simulink model "Sim48"  (R2019a)
settings: Solver=FixedStepAuto  StartTime=0.0  StopTime=10.0  FixedStep=0.0001  RelTol=1e-3
settings Model: Creator=fbleo  LastModifiedBy=fbleo

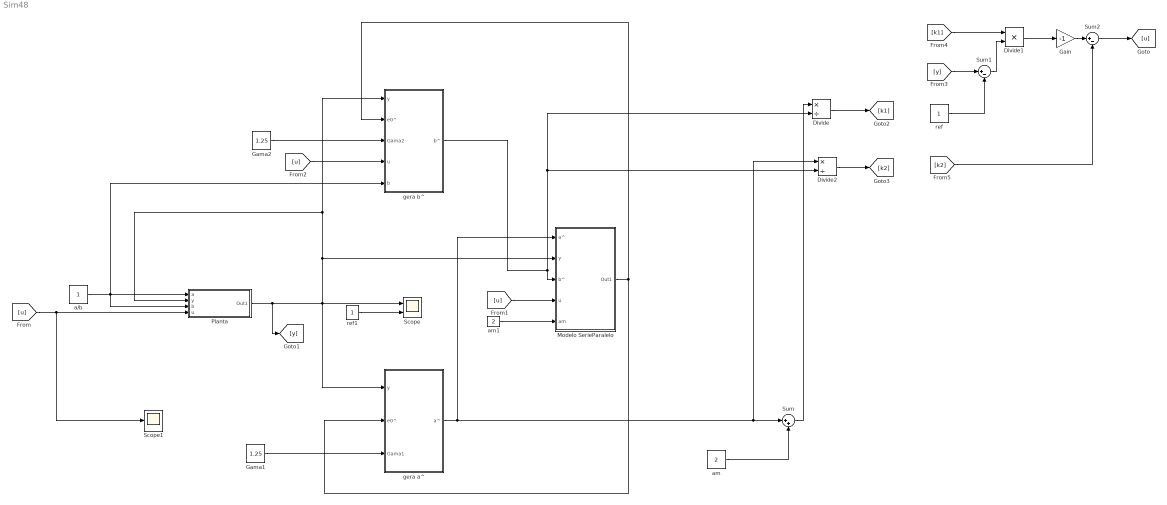
== system Sim48 ==
  Divide : Product  Inputs=*/
  Divide1 : Product  Inputs=**
  Divide2 : Product  Inputs=*/
  Gain : Gain  Gain=-1
  Gama1 : Constant  Value=1.25
  Gama2 : Constant  Value=1.25
  Modelo SerieParalelo : Subsystem
  Planta : Subsystem
  Scope : Scope  NumInputPorts=2
  Scope1 : Scope
  Sum : Sum  Inputs=|++
  Sum1 : Sum  Inputs=|+-
  Sum2 : Sum  Inputs=|+-
  a/b : Constant
  am : Constant  Value=2
  am1 : Constant  Value=2
  gera a^ : Subsystem
  gera b^ : Subsystem
  ref : Constant
  ref1 : Constant
  wires:
  Gama1/1 -> gera a^/3("Gama1 ")
  Divide1/1 -> Gain/1
  Gama2/1 -> gera b^/3("Gama2 ")
  [u] -> gera b^/4(u)
  Planta/1(Out1) -> [y], gera a^/1(y), gera b^/1(y), Planta/2(y), Modelo SerieParalelo/2(y), Scope/1
  am1/1 -> Modelo SerieParalelo/5(am)
  a/b/1 -> gera b^/5(b), Planta/3(b), Planta/1(a)
  Modelo SerieParalelo/1(Out1) -> gera a^/2(e0^), gera b^/2(e0^)
  gera b^/1(b^) -> Divide2/2, Divide/2, Modelo SerieParalelo/3(b^)
  [u] -> Scope1/1, Planta/4(u)
  gera a^/1(a^) -> Divide2/1, Sum/1, Modelo SerieParalelo/1(a^)
  am/1 -> Sum/2
  [u] -> Modelo SerieParalelo/4(u)
  Sum/1 -> Divide/1
  Divide/1 -> [k1]
  Divide2/1 -> [k2]
  [k1] -> Divide1/1
  [y] -> Sum1/1
  ref/1 -> Sum1/2
  Sum1/1 -> Divide1/2
  Gain/1 -> Sum2/1
  [k2] -> Sum2/2
  Sum2/1 -> [u]
  ref1/1 -> Scope/2

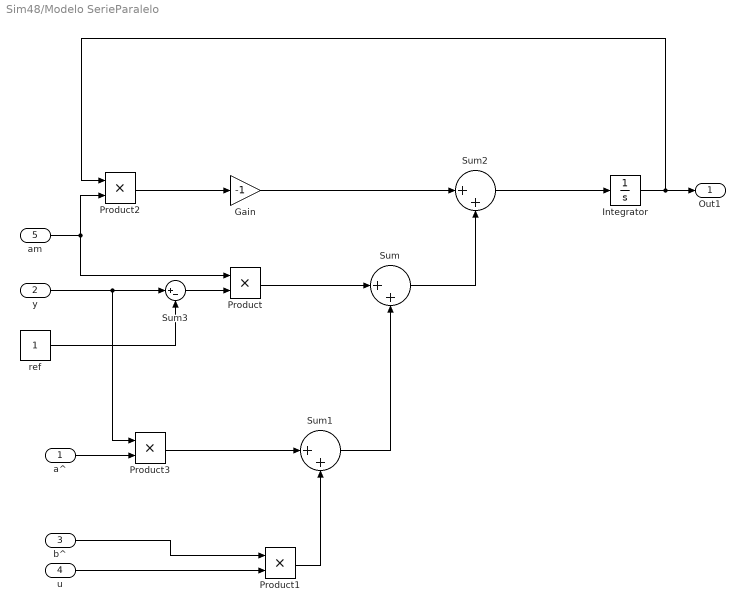
== system Sim48/Modelo SerieParalelo ==
  a^ : Inport
  y : Inport  Port=2
  b^ : Inport  Port=3
  u : Inport  Port=4
  am : Inport  Port=5
  Gain : Gain  Gain=-1
  Integrator : Integrator  InitialCondition=1.25
  Product{,1..3} (4 alike) : Product
  Sum : Sum  Inputs=|++
  Sum1 : Sum  Inputs=|++
  Sum2 : Sum  Inputs=|++
  Sum3 : Sum  Inputs=|+-
  ref : Constant
  Out1 : Outport
  wires:
  Product/1 -> Sum/1
  u/1 -> Product1/2
  b^/1 -> Product1/1
  Product1/1 -> Sum1/2
  Sum/1 -> Sum2/2
  Integrator/1 -> Product2/1, Out1/1
  am/1 -> Product/1, Product2/2
  Product2/1 -> Gain/1
  Gain/1 -> Sum2/1
  Sum2/1 -> Integrator/1
  ref/1 -> Sum3/2
  y/1 -> Product3/1, Sum3/1
  Sum3/1 -> Product/2
  a^/1 -> Product3/2
  Product3/1 -> Sum1/1
  Sum1/1 -> Sum/2

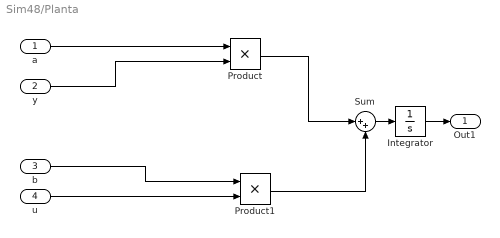
== system Sim48/Planta ==
  a : Inport
  y : Inport  Port=2
  b : Inport  Port=3
  u : Inport  Port=4
  Integrator : Integrator  InitialCondition=0.5
  Product : Product
  Product1 : Product
  Sum : Sum  Inputs=|++
  Out1 : Outport
  wires:
  a/1 -> Product/1
  y/1 -> Product/2
  Product/1 -> Sum/1
  u/1 -> Product1/2
  b/1 -> Product1/1
  Product1/1 -> Sum/2
  Sum/1 -> Integrator/1
  Integrator/1 -> Out1/1

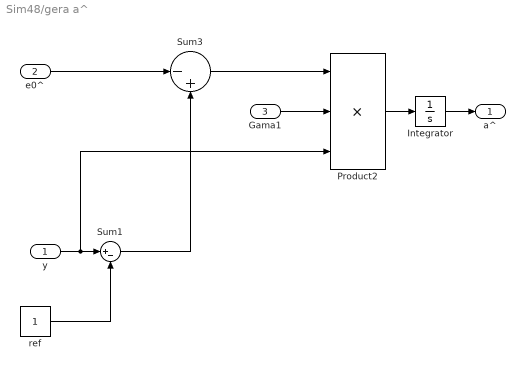
== system Sim48/gera a^ ==
  y : Inport
  e0^ : Inport  Port=2
  "Gama1 " : Inport  Port=3
  Integrator : Integrator  InitialCondition=0.7
  Product2 : Product  Inputs=3
  Sum1 : Sum  Inputs=|+-
  Sum3 : Sum  Inputs=|-+
  ref : Constant
  a^ : Outport
  wires:
  Sum3/1 -> Product2/1
  e0^/1 -> Sum3/1
  "Gama1 "/1 -> Product2/2
  Integrator/1 -> a^/1
  Product2/1 -> Integrator/1
  y/1 -> Product2/3, Sum1/1
  ref/1 -> Sum1/2
  Sum1/1 -> Sum3/2

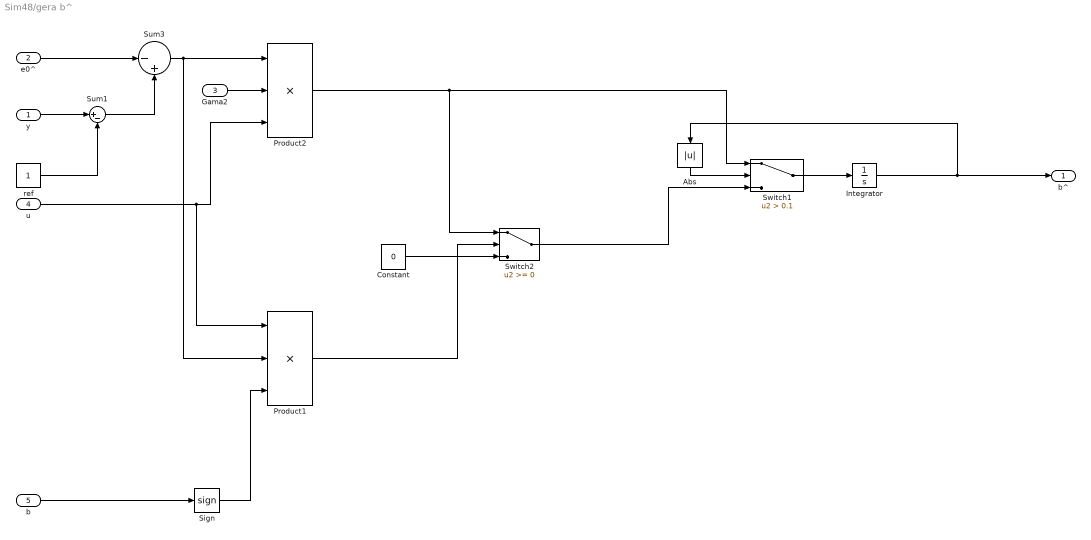
== system Sim48/gera b^ ==
  y : Inport
  e0^ : Inport  Port=2
  "Gama2 " : Inport  Port=3
  u : Inport  Port=4
  b : Inport  Port=5
  Abs : Abs
  Constant : Constant  Value=0
  Integrator : Integrator  InitialCondition=0.7
  Product1 : Product  Inputs=3
  Product2 : Product  Inputs=3
  Sign : Signum
  Sum1 : Sum  Inputs=|+-
  Sum3 : Sum  Inputs=|-+
  Switch1 : Switch  Criteria=u2 > Threshold  Threshold=0.1
  Switch2 : Switch
  ref : Constant
  b^ : Outport
  wires:
  Sum3/1 -> Product1/2, Product2/1
  e0^/1 -> Sum3/1
  "Gama2 "/1 -> Product2/2
  u/1 -> Product2/3, Product1/1
  Integrator/1 -> Abs/1, b^/1
  b/1 -> Sign/1
  Sign/1 -> Product1/3
  Product2/1 -> Switch2/1, Switch1/1
  Abs/1 -> Switch1/2
  Product1/1 -> Switch2/2
  Constant/1 -> Switch2/3
  Switch2/1 -> Switch1/3
  Switch1/1 -> Integrator/1
  ref/1 -> Sum1/2
  y/1 -> Sum1/1
  Sum1/1 -> Sum3/2
